simulink model "SimuTCP"  (R2022b)
settings: Solver=VariableStepAuto  StartTime=0.0  StopTime=inf  RelTol=1e-3
undefined symbols (not defined in the file): LF
libraries: instrumentseriallib x3, prociolib x3, instrumentlib x2, svdutilitieslib x1
settings Model: Creator=Jovani  LastModifiedBy=Jovani

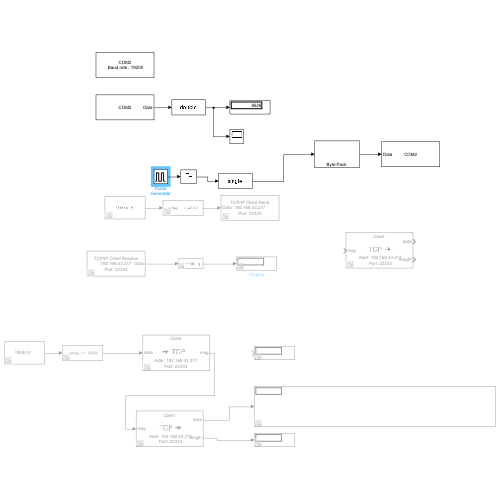
[thumbnail: Simulink's stored preview of the top-level diagram]
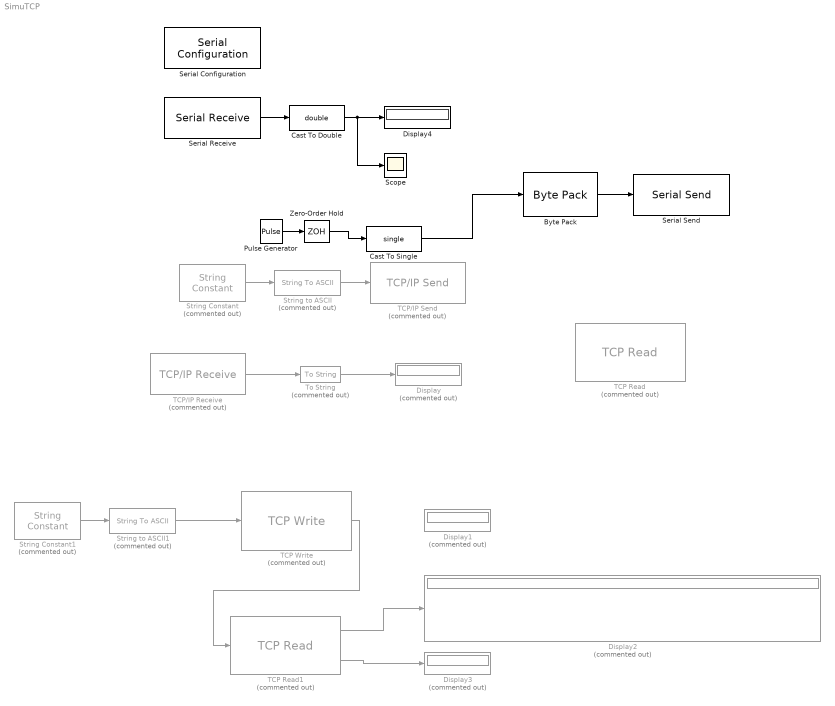
== system SimuTCP ==
  Byte Pack : svdutilitieslib/Byte Pack  maskPackedDataType=uint32  datatypes={'single'}  byteAlign=4  blockPlatform=arduinoert
  Cast To Double : DataTypeConversion  OutDataTypeStr=double  SaturateOnIntegerOverflow=off  RndMeth=Floor
  Cast To Single : DataTypeConversion  OutDataTypeStr=single  SaturateOnIntegerOverflow=off  RndMeth=Floor
  Display{,1..3} (4 alike) : Display  Commented=on
  Display4 : Display
  Pulse Generator : DiscretePulseGenerator  PulseType=Time based  Period=1  PulseWidth=5
  Scope : Scope
  Serial Configuration : instrumentseriallib/Serial Configuration  Priority=-200000  PortSel=COM2  Port=COM2  ComPort=COM2  BaudRate=19200  DataBits=8  Parity=none  StopBits=1  ByteOrder=little-endian  FlowControl=none  Timeout=10  SimulateUsing=Interpreted execution  BlockInModel=on  aMode=1
  Serial Receive : instrumentseriallib/Serial Receive  Priority=1  PortSel=COM2  Port=COM2  ComPort=COM2  DataType=single  SaveDataType=uint8  ToggleHeader=on  Header='x'  ToggleTerminator=on  Terminator=LF ('\n')  CustomTerminator=[]  InputFormat=Column major  ToggleDataSize=on  DataSize=[1 1]  EnableBlockingMode=on  ActionDataUnavailable=Output last received value  ActionWhenDataUnavailable=Output last received value  CustomValue=0  SampleTime=0.01  SimulateUsing=Interpreted execution  BlockInModel=on  aMode=1
  Serial Send : instrumentseriallib/Serial Send  Priority=1  PortSel=COM2  Port=COM2  ComPort=COM2  Header=[]  Terminator=<none>  CustomTerminator=[]  EnableBlockingMode=on  SimulateUsing=Interpreted execution  BlockInModel=on  aMode=1
  String Constant : StringConstant  Commented=on  String="\"Hello! r\""
  String Constant1 : StringConstant  Commented=on  String="\"Hello! r\""
  String to ASCII : StringToASCII  Commented=on
  String to ASCII1 : StringToASCII  Commented=on
  TCP Read : prociolib/TCP Read  Commented=on  NetworkRole=Client  RemoteAddress=192.168.43.217  RemotePort=22333  LocalPort=-1  DataType=uint8  DataLength=1  ByteOrder=LittleEndian  EnableEvent=off  OutputVarSizeSignal=off  OutputStatus=off  SampleTime=-1  hoistedMaskSrc=Variant/CODEGEN/TCP Read
  TCP Read1 : prociolib/TCP Read  Commented=on  NetworkRole=Client  RemoteAddress=192.168.43.217  RemotePort=22333  LocalPort=-1  DataType=uint8  DataLength=31  ByteOrder=LittleEndian  EnableEvent=off  OutputVarSizeSignal=off  OutputStatus=off  SampleTime=-1  hoistedMaskSrc=Variant/CODEGEN/TCP Read
  TCP Write : prociolib/TCP Write  Commented=on  NetworkRole=Client  RemoteAddress=192.168.43.217  RemotePort=22333  LocalPort=-1  ByteOrder=LittleEndian  OutputStatus=off  hoistedMaskSrc=Variant/CODEGEN/TCP Write
  TCP/IP Receive : instrumentlib/TCP//IP Receive  Commented=on  Host=192.168.43.217  Port=22333  DataSize=[ 1, 1 ]  DataType=ASCII  ASCIIFormatting=%f  Terminator=LF  CustomTerminator=10  ByteOrder=big-endian  EnableBlockingMode=on  Timeout=10  SampleTime=0.01  SimulateUsing=Interpreted execution
  TCP/IP Send : instrumentlib/TCP//IP Send  Commented=on  Host=192.168.43.217  Port=22333  ByteOrder=little-endian  EnableBlockingMode=on  Timeout=10  TransferDelay=on  SimulateUsing=Interpreted execution
  To String : ToString  Commented=on
  Zero-Order Hold : ZeroOrderHold  SampleTime=-1
  wires:
  String Constant/1 -> String to ASCII/1
  String to ASCII/1 -> TCP/IP Send/1
  To String/1 -> Display/1
  TCP/IP Receive/1 -> To String/1
  String Constant1/1 -> String to ASCII1/1
  String to ASCII1/1 -> TCP Write/1
  TCP Write/1 -> TCP Read1/1
  TCP Read1/1 -> Display2/1
  TCP Read1/2 -> Display3/1
  Serial Receive/1 -> Cast To Double/1
  Cast To Double/1 -> Scope/1, Display4/1
  Byte Pack/1 -> Serial Send/1
  Cast To Single/1 -> Byte Pack/1
  Zero-Order Hold/1 -> Cast To Single/1
  Pulse Generator/1 -> Zero-Order Hold/1
